simulink model "ABB_1010"  (R2024a)
settings: Solver=VariableStepAuto  StartTime=0.0  StopTime=200  RelTol=1e-3
model workspace: external: MATLAB File C:\Users\lucas\OneDrive\Documents\MATLAB\projeto final\ABB_1010_DataFile.m (data not in the file)
values from neighbouring files (symbols this model uses):
  g = 9.81    [inicializacaoAntropomorfico.m]
  I1 = [ 0.00243841  0.00000307  0.00007261    [inicializacaoAntropomorfico.m]
  I2 = [ 0.01633569  0.00000387 -0.00034405    [inicializacaoAntropomorfico.m]
  I3 = [ 0.00244760 -0.00000208  0.00000538    [inicializacaoAntropomorfico.m]
  I4 = [ 0.00245792 -0.00000008  0.00003121    [inicializacaoAntropomorfico.m]
  I5 = [ 0.00062165 -0.00000206 -0.00000303    [inicializacaoAntropomorfico.m]
  I6 = [ 0.00000357  0.00000000  0.00000000    [inicializacaoAntropomorfico.m]
  I7 = [(m7*L7^2)/12 0.00000000  0.00000000    [inicializacaoAntropomorfico.m]
  L = [L1, L2, L3, L4, L5, L6, L7]    [inicializacaoAntropomorfico.m]
  Lcm1 = [-0.00258308  0.00024508 -0.01434968]    [inicializacaoAntropomorfico.m]
  Lcm2 = [-0.02078894  0.00020016 -0.10516734]    [inicializacaoAntropomorfico.m]
  Lcm3 = [ 0.00021912  0.00015355 -0.06228290]    [inicializacaoAntropomorfico.m]
  Lcm4 = [-0.00172658 -0.00124140 -0.07369196]    [inicializacaoAntropomorfico.m]
  Lcm5 = [-0.00014110  0.00085992 -0.03825278]    [inicializacaoAntropomorfico.m]
  Lcm6 = [ 0.00002478  0.00000000 -0.00042157]    [inicializacaoAntropomorfico.m]
  Lcm7 = [ 0           0          -0.05000000]    [inicializacaoAntropomorfico.m]
  m = [m1, m2, m3, m4, m5, m6, m7]    [inicializacaoAntropomorfico.m]
  Pf = [  0.05    [inicializacaoAntropomorfico.m]
  Pi = [  0.2    [inicializacaoAntropomorfico.m]
  Raio = [0]    [inicializacaoAntropomorfico.m]
  Sentido = [0]    [inicializacaoAntropomorfico.m]
  Tipo = [1]    [inicializacaoAntropomorfico.m]
undefined symbols (not defined in the file or in its folder): smiData, X, Y, Z
libraries: sm_lib x35, nesl_utility x7
(part 3 of 16)

== matlab function ABB_1010/Dinamica1/MATLAB Function1 ==
  data: I1 parameter; L parameter; Lcm1 parameter; H output; Q input; I2 parameter; I3 parameter; I4 parameter; I5 parameter; I6 parameter; Lcm2 parameter; Lcm3 parameter; Lcm4 parameter; Lcm5 parameter; Lcm6 parameter; dQ input; m parameter; Lcm7 parameter; I7 parameter
function H = func_H(I1, L, Lcm1, Q, I2, I3, I4, I5, I6, Lcm2, Lcm3, Lcm4, Lcm5, Lcm6, dQ, m, Lcm7, I7)
%func_H
%    OUT1 = func_H(Ixx2,Ixx3,Ixx4,Ixx5,Ixx6,Ixy2,Ixy3,Ixy4,Ixy5,Ixy6,Ixz2,Ixz3,Ixz4,Ixz5,Ixz6,Iyx2,Iyx3,Iyx4,Iyx5,Iyx6,Iyy4,Iyy5,Iyy6,Iyz2,Iyz3,Iyz4,Iyz5,Iyz6,Izx2,Izx3,Izx4,Izx5,Izx6,Izy2,Izy3,Izy4,Izy5,Izy6,Izz2,Izz3,Izz4,Izz5,Izz6,Lx2,Lx3,Lxcm2,Lxcm3,Lxcm4,Lxcm5,Lxcm6,Lycm2,Lycm3,Lycm4,Lycm5,Lycm6,Lz4,Lz5,Lzcm2,Lzcm3,Lzcm4,Lzcm5,Lzcm6,Q1,Q2,Q3,Q4,Q5,Q6,dQ1,dQ2,dQ3,dQ4,dQ5,dQ6,M2,M3,M4,M5,M6)

%    This function was generated by the Symbolic Math Toolbox version 24.1.
%    30-Apr-2025 06:22:27
H   = zeros(6,1);
m1  = m(1);
m2  = m(2);
m3  = m(3);
m4  = m(4);
m5  = m(5);
m6  = m(6);
m7  = m(7);

Q1  = Q(1);
Q2  = Q(2);
Q3  = Q(3);
Q4  = Q(4);
Q5  = Q(5);
Q6  = Q(6);

dQ1  = dQ(1);
dQ2  = dQ(2);
dQ3  = dQ(3);
dQ4  = dQ(4);
dQ5  = dQ(5);
dQ6  = dQ(6);

Lz1 = L(1);
Lx2 = L(2);
Lx3 = L(3);
Lx4 = L(4);
Lz5 = L(5);
Lz6 = L(6);
Lz7 = L(7);

Lxcm1 = Lcm1(1);
Lycm1 = Lcm1(2);
Lzcm1 = Lcm1(3);

Lxcm2 = Lcm2(1);
Lycm2 = Lcm2(2);
Lzcm2 = Lcm2(3);

Lxcm3 = Lcm3(1);
Lycm3 = Lcm3(2);
Lzcm3 = Lcm3(3);

Lxcm4 = Lcm4(1);
Lycm4 = Lcm4(2);
Lzcm4 = Lcm4(3);

Lxcm5 = Lcm5(1);
Lycm5 = Lcm5(2);
Lzcm5 = Lcm5(3);

Lxcm6 = Lcm6(1);
Lycm6 = Lcm6(2);
Lzcm6 = Lcm6(3);

Lxcm7 = Lcm7(1);
Lycm7 = Lcm7(2);
Lzcm7 = Lcm7(3);

Ixx1 = I1(1,1);
Ixy1 = I1(1,2);
Ixz1 = I1(1,3);
Iyx1 = I1(2,1);
Iyy1 = I1(2,2);
Iyz1 = I1(2,3);
Izx1 = I1(3,1);
Izy1 = I1(3,2);
Izz1 = I1(3,3);

Ixx2 = I2(1,1);
Ixy2 = I2(1,2);
Ixz2 = I2(1,3);
Iyx2 = I2(2,1);
Iyy2 = I2(2,2);
Iyz2 = I2(2,3);
Izx2 = I2(3,1);
Izy2 = I2(3,2);
Izz2 = I2(3,3);

Ixx3 = I3(1,1);
Ixy3 = I3(1,2);
Ixz3 = I3(1,3);
Iyx3 = I3(2,1);
Iyy3 = I3(2,2);
Iyz3 = I3(2,3);
Izx3 = I3(3,1);
Izy3 = I3(3,2);
Izz3 = I3(3,3);

Ixx4 = I4(1,1);
Ixy4 = I4(1,2);
Ixz4 = I4(1,3);
Iyx4 = I4(2,1);
Iyy4 = I4(2,2);
Iyz4 = I4(2,3);
Izx4 = I4(3,1);
Izy4 = I4(3,2);
Izz4 = I4(3,3);

Ixx5 = I5(1,1);
Ixy5 = I5(1,2);
Ixz5 = I5(1,3);
Iyx5 = I5(2,1);
Iyy5 = I5(2,2);
Iyz5 = I5(2,3);
Izx5 = I5(3,1);
Izy5 = I5(3,2);
Izz5 = I5(3,3);

Ixx6 = I6(1,1);
Ixy6 = I6(1,2);
Ixz6 = I6(1,3);
Iyx6 = I6(2,1);
Iyy6 = I6(2,2);
Iyz6 = I6(2,3);
Izx6 = I6(3,1);
Izy6 = I6(3,2);
Izz6 = I6(3,3);

Ixx7 = I7(1,1);
Ixy7 = I7(1,2);
Ixz7 = I7(1,3);
Iyx7 = I7(2,1);
Iyy7 = I7(2,2);
Iyz7 = I7(2,3);
Izx7 = I7(3,1);
Izy7 = I7(3,2);
Izz7 = I7(3,3);


t2 = cos(Q1);
t3 = cos(Q2);
t4 = cos(Q3);
t5 = cos(Q4);
t6 = cos(Q5);
t7 = cos(Q6);
t8 = sin(Q1);
t9 = sin(Q2);
t10 = sin(Q3);
t11 = sin(Q4);
t12 = sin(Q5);
t13 = sin(Q6);
t14 = Q2+Q3;
t15 = Lx4^2;
t16 = Lxcm4^2;
t17 = Lxcm5^2;
t18 = Lxcm6^2;
t19 = Lycm4^2;
t20 = Lycm5^2;
t21 = Lycm6^2;
t22 = Lz6^2;
t23 = Lzcm5^2;
t24 = Lzcm6^2;
t25 = Q2*2.0;
t27 = Q4*2.0;
t28 = Q5*2.0;
t29 = Q6*2.0;
t30 = dQ1^2;
t31 = dQ2^2;
t32 = dQ3^2;
t33 = dQ4^2;
t34 = dQ5^2;
t35 = dQ6^2;
t36 = cos(t27);
t37 = cos(t28);
t38 = cos(t29);
t39 = t5^2;
t40 = t6^2;
t41 = t7^2;
t42 = sin(t25);
t43 = t11^2;
t44 = t12^2;
t45 = t13^2;
t46 = Lycm3*t2;
t47 = Lzcm2*t3;
t48 = cos(t14);
t49 = Lx2*t9;
t50 = Lxcm2*t9;
t51 = Lycm3*t8;
t52 = sin(t14);
t53 = t2*t5;
t54 = Lzcm3*m3*t4;
t55 = Lzcm4*m4*t4;
t56 = t2*t11;
t57 = t5*t8;
t58 = Lx3*m3*t10;
t59 = Lx3*m4*t10;
t60 = Lx3*m5*t10;
t61 = Lx3*m6*t10;
t62 = Lxcm3*m3*t10;
t63 = t8*t11;
t65 = Lx2*t2*t3;
t68 = Lzcm4*t3*t4;
t69 = Lx3*Lycm4*m4*t5;
t70 = Lx3*Lycm5*m5*t5;
t71 = Lx3*Lz6*m6*t6;
t72 = Lx4*Lzcm4*m4*t5;
t73 = Lx3*Lzcm5*m5*t6;
t74 = Lx3*Lzcm6*m6*t6;
t75 = Lxcm4*Lzcm4*m4*t5;
t76 = Lxcm5*Lzcm5*m5*t5;
t79 = Ixx4*t5*t11;
t80 = Ixx6*t5*t11;
t81 = Ixx5*t6*t12;
t82 = Ixx6*t7*t13;
t83 = Iyy4*t5*t11;
t84 = Iyy5*t5*t11;
t85 = Iyy6*t6*t12;
t86 = Iyy6*t7*t13;
t87 = Izz5*t5*t11;
t88 = Izz6*t5*t11;
t89 = Izz5*t6*t12;
t90 = Izz6*t6*t12;
t91 = Lx2*t3*t8;
t92 = Lx3*t3*t10;
t93 = Lx3*t4*t9;
t98 = Lx3*Lx4*m4*t11;
t99 = Lx3*Lx4*m5*t11;
t100 = Lx3*Lx4*m6*t11;
t101 = Lx3*Lxcm4*m4*t11;
t102 = Lx3*Lxcm5*m5*t12;
t103 = Lycm4*Lzcm4*m4*t11;
t106 = Lzcm4*t9*t10;
t110 = Lxcm6*Lz6*t5*t7;
t111 = Lxcm6*Lzcm6*t5*t7;
t112 = Lx3*Lxcm6*t7*t12;
t113 = Lycm6*Lz6*t5*t13;
t114 = Lycm6*Lzcm6*t5*t13;
t116 = t2*t3*t4;
t117 = Lx3*Lycm6*t12*t13;
t118 = Lz6*m6*t4*t6;
t119 = Lzcm5*m5*t4*t6;
t120 = Lzcm6*m6*t4*t6;
t123 = t2*t3*t10;
t124 = t2*t4*t9;
t125 = t3*t4*t8;
t127 = Lx4*m4*t5*t10;
t128 = Lx4*m5*t5*t10;
t129 = Lx4*m6*t5*t10;
t130 = Lxcm4*m4*t5*t10;
t131 = Lxcm5*m5*t4*t12;
t133 = t2*t9*t10;
t134 = t3*t8*t10;
t135 = t4*t8*t9;
t137 = Lycm4*m4*t10*t11;
t138 = Lycm5*m5*t10*t11;
t139 = t8*t9*t10;
t140 = t14*2.0;
t170 = Lx3*Lycm6*m6*t5*t7;
t172 = Lx4*Lz6*m6*t5*t6;
t174 = Lx4*Lzcm5*m5*t5*t6;
t176 = Lx4*Lzcm6*m6*t5*t6;
t187 = Lx4*t3*t5*t10;
t188 = Lx4*t4*t5*t9;
t190 = Lxcm4*t3*t5*t10;
t191 = Lxcm4*t4*t5*t9;
t199 = Lx3*Lxcm5*m5*t6*t11;
t200 = Lx4*Lxcm5*m5*t5*t12;
t201 = Lx3*Lxcm6*m6*t5*t13;
t202 = Lx3*Lxcm6*m6*t7*t11;
t205 = Lycm6*Lz6*m6*t7*t12;
t206 = Lycm5*Lzcm5*m5*t6*t11;
t208 = Lycm6*Lzcm6*m6*t7*t12;
t214 = Lycm4*t3*t10*t11;
t215 = Lycm4*t4*t9*t11;
t221 = Lx3*Lycm6*m6*t11*t13;
t223 = Lxcm5*Lycm5*m5*t11*t12;
t224 = Lxcm6*Lycm6*m6*t11*t12;
t225 = Lx3*Lz6*m6*t11*t12;
t226 = Lx3*Lzcm5*m5*t11*t12;
t227 = Lx3*Lzcm6*m6*t11*t12;
t228 = Lxcm6*Lz6*m6*t12*t13;
t229 = Lxcm6*Lzcm6*m6*t12*t13;
t235 = Lx4*Lxcm6*t5*t7*t12;
t236 = Lycm6*Lz6*t6*t7*t11;
t237 = Lycm6*Lzcm6*t6*t7*t11;
t239 = Lx4*Lycm6*t5*t12*t13;
t240 = Lxcm6*Lz6*t6*t11*t13;
t241 = Lxcm6*Lzcm6*t6*t11*t13;
t247 = Lxcm5*m5*t5*t6*t10;
t248 = Lxcm6*m6*t4*t7*t12;
t256 = Lycm6*m6*t7*t10*t11;
t257 = Lycm6*m6*t4*t12*t13;
t258 = Lz6*m6*t5*t10*t12;
t259 = Lzcm5*m5*t5*t10*t12;
t260 = Lzcm6*m6*t5*t10*t12;
t267 = Lxcm6*m6*t10*t11*t13;
t278 = Lx4*Lxcm4*m4*t5*t11*2.0;
t279 = Lz6*Lzcm6*m6*t5*t11*2.0;
t280 = Lz6*Lzcm6*m6*t6*t12*2.0;
t281 = m4*t5*t11*t15;
t282 = m5*t5*t11*t15;
t283 = m6*t5*t11*t15;
t284 = m4*t5*t11*t16;
t285 = m5*t6*t12*t17;
t286 = m6*t5*t11*t18;
t287 = m6*t7*t13*t18;
t288 = m4*t5*t11*t19;
t289 = m5*t5*t11*t20;
t290 = m6*t6*t12*t21;
t291 = m6*t7*t13*t21;
t292 = m6*t5*t11*t22;
t293 = m6*t6*t12*t22;
t294 = m5*t5*t11*t23;
t295 = m5*t6*t12*t23;
t296 = m6*t5*t11*t24;
t297 = m6*t6*t12*t24;
t352 = Lx4*Lxcm6*m6*t5*t7*t11;
t374 = Lx4*Lycm6*m6*t5*t11*t13;
t420 = Lycm6*m6*t5*t6*t10*t13;
t434 = Lx4*Lxcm5*m5*t5*t6*t11*2.0;
t436 = Lx4*Lz6*m6*t5*t11*t12*2.0;
t437 = Lx4*Lzcm5*m5*t5*t11*t12*2.0;
t438 = Lx4*Lzcm6*m6*t5*t11*t12*2.0;
t453 = Lxcm6*m6*t5*t6*t7*t10;
t590 = Lxcm6*Lycm6*m6*t5*t7*t11*t13*2.0;
t591 = Lxcm6*Lycm6*m6*t6*t7*t12*t13*2.0;
t679 = Lxcm6*Lycm6*m6*t5*t6*t7*t11*t13*4.0;
t64 = Lzcm3*t48;
t66 = Lycm4*t53;
t67 = Lycm5*t53;
t77 = Lx3*t52;
t78 = Lxcm3*t52;
t94 = Lx4*t56;
t95 = Lxcm4*t56;
t96 = Lycm4*t57;
t97 = Lycm5*t57;
t104 = Lx4*t63;
t105 = Lxcm4*t63;
t107 = -t47;
t108 = -t51;
t109 = t52^2;
t115 = t6*t48;
t121 = t12*t48;
t122 = t6*t52;
t126 = t6*t56;
t132 = t12*t52;
t136 = t12*t56;
t141 = -t53;
t142 = -t54;
t143 = -t55;
t144 = -t63;
t146 = -t65;
t147 = -t68;
t148 = -t76;
t149 = -t79;
t150 = -t87;
t151 = -t88;
t152 = -t89;
t153 = -t90;
t155 = -t103;
t156 = sin(t140);
t159 = Lx4*Lycm4*m4*t36;
t160 = Lx4*Lycm5*m5*t36;
t161 = Lxcm4*Lycm4*m4*t36;
t162 = Lxcm6*Lycm6*m6*t38;
t163 = Lxcm5*Lzcm5*m5*t37;
t164 = Lx3*t2*t48;
t168 = Lx3*t116;
t169 = Lxcm3*t116;
t171 = t5*t71;
t173 = t5*t73;
t175 = t5*t74;
t177 = m6*t110;
t178 = m6*t111;
t179 = Lx3*t8*t48;
t180 = Lx4*t5*t52;
t182 = t5*t81;
t183 = t5*t85;
t186 = Lx3*t125;
t189 = Lxcm3*t125;
t193 = Lycm6*t7*t57;
t194 = Lzcm3*t123;
t195 = Lzcm3*t124;
t196 = Lzcm4*t123;
t197 = Lzcm4*t124;
t198 = t5*t102;
t203 = m6*t112;
t204 = m6*t113;
t207 = m6*t114;
t209 = Lycm5*t11*t52;
t210 = Lx3*t133;
t211 = Lxcm3*t133;
t212 = Lxcm5*t6*t63;
t213 = Lxcm6*t13*t57;
t216 = Lzcm3*t134;
t217 = Lzcm3*t135;
t218 = Lzcm4*t134;
t219 = Lzcm4*t135;
t222 = m6*t117;
t230 = Lx3*t139;
t231 = Lxcm3*t139;
t232 = Lz6*t12*t63;
t233 = Lzcm5*t12*t63;
t234 = Lzcm6*t12*t63;
t244 = t7*t11*t48;
t246 = t3*t4*t57;
t251 = t11*t13*t48;
t252 = t7*t11*t52;
t262 = t11*t13*t52;
t264 = t9*t10*t57;
t265 = -t110;
t266 = -t111;
t268 = t9*t10*t63;
t269 = -t112;
t270 = -t118;
t271 = -t119;
t272 = -t120;
t274 = -t133;
t275 = -t137;
t276 = -t138;
t277 = -t139;
t298 = Lx4*Lycm6*m6*t7*t39;
t299 = Lxcm5*Lycm5*m5*t6*t39;
t300 = Lxcm6*Lycm6*m6*t6*t39;
t301 = Lx4*Lz6*m6*t6*t39;
t302 = Lx4*Lzcm5*m5*t6*t39;
t303 = Lx4*Lzcm6*m6*t6*t39;
t304 = Lxcm6*Lz6*m6*t7*t40;
t305 = Lxcm6*Lzcm6*m6*t7*t40;
t306 = Ixx5*t5*t11*t40;
t307 = t39*t81;
t308 = t41*t80;
t309 = Ixx6*t6*t12*t41;
t310 = t39*t82;
t311 = t40*t82;
t312 = Iyy6*t5*t11*t40;
t313 = Iyy6*t5*t11*t41;
t314 = t39*t85;
t315 = t41*t85;
t316 = t39*t86;
t317 = t40*t86;
t318 = t40*t87;
t319 = t39*t89;
t320 = t40*t88;
t321 = t39*t90;
t322 = Lx4*Lxcm5*m5*t12*t39;
t323 = Lx4*Lxcm6*m6*t13*t39;
t324 = Lx4*Lycm6*m6*t7*t43;
t325 = Lxcm5*Lycm5*m5*t6*t43;
t326 = Lxcm6*Lycm6*m6*t6*t43;
t327 = Lxcm6*Lz6*m6*t7*t44;
t328 = Lxcm6*Lzcm6*m6*t7*t44;
t329 = Lycm6*Lz6*m6*t13*t40;
t330 = Lycm5*Lzcm5*m5*t12*t39;
t331 = Lycm6*Lzcm6*m6*t13*t40;
t332 = Lx4*Lxcm6*m6*t13*t43;
t333 = Lycm6*Lz6*m6*t13*t44;
t334 = Lycm5*Lzcm5*m5*t12*t43;
t335 = Lycm6*Lzcm6*m6*t13*t44;
t336 = Lx4*t3*t4*t53;
t337 = Lxcm4*t3*t4*t53;
t338 = t6*t170;
t346 = Lycm4*t3*t4*t56;
t347 = Lycm5*t3*t4*t56;
t348 = Lx2*t247;
t349 = t6*t201;
t351 = t6*t202;
t353 = m6*t235;
t354 = m6*t236;
t355 = t6*t205;
t356 = t5*t206;
t357 = m6*t237;
t358 = t6*t208;
t365 = Lx4*t9*t10*t53;
t367 = Lxcm5*t12*t123;
t368 = Lxcm5*t12*t124;
t369 = Lxcm6*t6*t7*t63;
t373 = t6*t221;
t375 = m6*t239;
t376 = t5*t223;
t377 = t5*t224;
t378 = Lx2*t258;
t379 = Lx2*t259;
t380 = Lx2*t260;
t381 = m6*t240;
t382 = t6*t228;
t383 = m6*t241;
t384 = t6*t229;
t387 = t11*t12*t82;
t388 = t11*t12*t86;
t391 = Lycm4*t9*t10*t56;
t392 = Lycm5*t9*t10*t56;
t407 = -t200;
t408 = -t206;
t412 = -t214;
t413 = -t215;
t414 = -t221;
t415 = -t224;
t423 = -t235;
t425 = t40*t76*2.0;
t428 = -t256;
t429 = -t257;
t433 = -t267;
t435 = t5*t280;
t439 = t5*t285;
t440 = t5*t290;
t441 = t5*t293;
t442 = t5*t295;
t443 = t5*t297;
t445 = -t285;
t446 = -t286;
t447 = -t288;
t448 = -t289;
t449 = -t290;
t454 = Lx4*Lycm6*m6*t12*t13*t39;
t455 = t39*t228;
t456 = t39*t229;
t457 = t43*t205;
t458 = t43*t208;
t459 = t43*t228;
t460 = t43*t229;
t482 = Lycm6*t3*t4*t7*t56;
t486 = Lx2*t453;
t492 = Lxcm5*t6*t9*t10*t53;
t493 = Lxcm6*t3*t4*t13*t56;
t494 = Lxcm6*t7*t12*t123;
t495 = Lxcm6*t7*t12*t124;
t497 = Lx2*t420;
t502 = t7*t12*t13*t80;
t505 = Lycm6*t7*t9*t10*t56;
t506 = Lycm6*t12*t13*t123;
t507 = Lycm6*t12*t13*t124;
t508 = Lz6*t9*t10*t12*t53;
t509 = Lzcm5*t9*t10*t12*t53;
t510 = Lzcm6*t9*t10*t12*t53;
t513 = Lxcm6*t9*t10*t13*t56;
t519 = Lxcm6*Lycm6*m6*t39*t41;
t520 = Lxcm6*Lycm6*m6*t40*t41;
t521 = Lxcm5*Lzcm5*m5*t39*t40;
t530 = Lxcm6*Lycm6*m6*t39*t45;
t531 = Lxcm6*Lycm6*m6*t40*t45;
t532 = Lxcm5*Lzcm5*m5*t39*t44;
t539 = -t374;
t560 = Lx4*Lxcm6*m6*t7*t12*t39;
t561 = t39*t205;
t562 = t39*t208;
t563 = t6*t45*t80;
t564 = t6*t43*t82;
t565 = Iyy6*t5*t6*t11*t45;
t566 = t6*t43*t86;
t567 = t41*t224*2.0;
t568 = m5*t5*t11*t17*t40;
t569 = t39*t285;
t570 = t41*t286;
t571 = m6*t6*t12*t18*t41;
t572 = t39*t287;
t573 = t40*t287;
t574 = m6*t5*t11*t21*t40;
t575 = m6*t5*t11*t21*t41;
t576 = t39*t290;
t577 = t41*t290;
t578 = t39*t291;
t579 = t40*t291;
t580 = t40*t292;
t581 = t39*t293;
t582 = t40*t294;
t583 = t39*t295;
t584 = t40*t296;
t585 = t39*t297;
t586 = -t420;
t588 = t6*t352*2.0;
t589 = t6*t374*2.0;
t592 = t6*t11*t12*t76*2.0;
t593 = t11*t12*t287;
t594 = t11*t12*t291;
t605 = t40*t279;
t611 = Lxcm6*t6*t7*t9*t10*t53;
t634 = -t590;
t648 = Ixx4*t39*t48*t52;
t650 = Iyy4*t43*t48*t52;
t651 = Iyy5*t43*t48*t52;
t663 = Lz6*Lzcm6*m6*t5*t11*t40*-2.0;
t664 = Lz6*Lzcm6*m6*t6*t12*t39*-2.0;
t665 = Lycm6*t3*t4*t6*t13*t53;
t678 = t5*t591;
t688 = t123+t124;
t690 = t134+t135;
t700 = t6*t43*t287;
t701 = m6*t5*t6*t11*t21*t45;
t702 = t6*t43*t291;
t703 = -t679;
t740 = Lxcm6*Lycm6*m6*t5*t7*t11*t13*t40*-2.0;
t145 = -t64;
t154 = -t96;
t157 = -t104;
t158 = -t105;
t165 = Lz6*t115;
t166 = Lzcm5*t115;
t167 = Lzcm6*t115;
t181 = Lxcm5*t121;
t192 = Lxcm5*t126;
t220 = Lzcm5*t136;
t238 = t5*t115;
t242 = t5*t121;
t243 = t5*t122;
t245 = t7*t121;
t249 = t8*t122;
t250 = t5*t132;
t253 = t13*t121;
t254 = t7*t132;
t261 = t8*t132;
t263 = t13*t132;
t341 = Lz6*t2*t122;
t342 = Lzcm5*t2*t122;
t343 = Lzcm6*t2*t122;
t344 = Lx4*t246;
t345 = Lxcm4*t246;
t350 = t5*t203;
t359 = Lycm6*t252;
t372 = t5*t222;
t386 = Lxcm6*t262;
t389 = Lx4*t264;
t390 = Lxcm4*t264;
t394 = Lycm4*t268;
t395 = Lycm5*t268;
t396 = -t164;
t400 = -t171;
t401 = -t173;
t402 = -t175;
t403 = -t177;
t404 = -t178;
t405 = t5*t152;
t406 = t5*t153;
t409 = -t209;
t410 = -t210;
t411 = -t211;
t416 = -t230;
t417 = -t231;
t419 = t12*t246;
out1 = ft_1({Ixx2,Ixx3,Ixx5,Ixx6,Iyy6,Izz2,Izz3,Izz4,Izz5,Izz6,Lx2,Lx3,Lx4,Lxcm2,Lxcm3,Lxcm4,Lxcm5,Lxcm6,Lycm2,Lycm3,Lycm4,Lycm5,Lycm6,Lz6,Lzcm2,Lzcm3,Lzcm4,Lzcm5,Lzcm6,m2,m3,m4,m5,m6,t10,t100,t101,t102,t104,t106,t107,t108,t109,t11,t113,t114,t115,t116,t117,t118,t119,t12,t120,t121,t122,t125,t126,t127,t128,t129,t13,t130,t131,t132,t136,t141,t142,t143,t144,t145,t146,t147,t148,t149,t150,t151,t152,t153,t154,t155,t156,t157,t158,t159,t160,t161,t162,t163,t165,t166,t167,t168,t169,t170,t172,t174,t176,t177,t178,t179,t180,t181,t182,t183,t186,t187,t188,t189,t190,t191,t192,t193,t194,t195,t196,t197,t198,t199,t2,t200,t201,t202,t203,t204,t205,t206,t207,t208,t212,t213,t216,t217,t218,t219,t220,t222,t223,t224,t225,t226,t227,t228,t229,t232,t233,t234,t236,t237,t238,t239,t240,t241,t242,t243,t244,t245,t246,t247,t248,t249,t250,t251,t252,t253,t254,t256,t257,t258,t259,t260,t261,t262,t263,t264,t265,t266,t268,t269,t270,t271,t272,t274,t275,t276,t277,t278,t279,t280,t281,t282,t283,t284,t285,t286,t287,t288,t289,t290,t291,t292,t293,t294,t295,t296,t297,t298,t299,t3,t30,t300,t301,t302,t303,t304,t305,t306,t307,t308,t309,t31,t310,t311,t312,t313,t314,t315,t316,t317,t318,t319,t32,t320,t321,t322,t323,t324,t325,t326,t327,t328,t329,t33,t330,t331,t332,t333,t334,t335,t336,t337,t338,t34,t341,t342,t343,t344,t345,t346,t347,t348,t349,t35,t350,t351,t352,t353,t354,t355,t356,t357,t358,t359,t365,t367,t368,t369,t372,t373,t374,t375,t376,t377,t378,t379,t380,t381,t382,t383,t384,t386,t387,t388,t389,t39,t390,t391,t392,t394,t395,t396,t4,t40,t400,t401,t402,t403,t404,t405,t406,t407,t408,t409,t41,t410,t411,t412,t413,t414,t415,t416,t417,t419,t42,t423,t425,t428,t429,t43,t433,t434,t435,t436,t437,t438,t439,t44,t440,t441,t442,t443,t445,t446,t447,t448,t449,t45,t453,t454,t455,t456,t457,t458,t459,t46,t460,t482,t486,t49,t492,t493,t494,t495,t497,t5,t50,t502,t505,t506,t507,t508,t509,t510,t513,t519,t52,t520,t521,t53,t530,t531,t532,t539,t54,t55,t56,t560,t561,t562,t563,t564,t565,t566,t567,t568,t569,t57,t570,t571,t572,t573,t574,t575,t576,t577,t578,t579,t58,t580,t581,t582,t583,t584,t585,t586,t588,t589,t59,t591,t592,t593,t594,t6,t60,t605,t61,t611,t62,t63,t634,t648,t65,t650,t651,t66,t663,t664,t665,t67,t678,t688,t69,t690,t7,t70,t700,t701,t702,t703,t71,t72,t73,t74,t740,t75,t76,t77,t78,t79,t8,t80,t81,t82,t83,t84,t85,t86,t87,t88,t89,t9,t90,t91,t92,t93,t94,t95,t97,t98,t99});
end
function out1 = ft_1(ct)
[Ixx2,Ixx3,Ixx5,Ixx6,Iyy6,Izz2,Izz3,Izz4,Izz5,Izz6,Lx2,Lx3,Lx4,Lxcm2,Lxcm3,Lxcm4,Lxcm5,Lxcm6,Lycm2,Lycm3,Lycm4,Lycm5,Lycm6,Lz6,Lzcm2,Lzcm3,Lzcm4,Lzcm5,Lzcm6,m2,m3,m4,m5,m6,t10,t100,t101,t102,t104,t106,t107,t108,t109,t11,t113,t114,t115,t116,t117,t118,t119,t12,t120,t121,t122,t125,t126,t127,t128,t129,t13,t130,t131,t132,t136,t141,t142,t143,t144,t145,t146,t147,t148,t149,t150,t151,t152,t153,t154,t155,t156,t157,t158,t159,t160,t161,t162,t163,t165,t166,t167,t168,t169,t170,t172,t174,t176,t177,t178,t179,t180,t181,t182,t183,t186,t187,t188,t189,t190,t191,t192,t193,t194,t195,t196,t197,t198,t199,t2,t200,t201,t202,t203,t204,t205,t206,t207,t208,t212,t213,t216,t217,t218,t219,t220,t222,t223,t224,t225,t226,t227,t228,t229,t232,t233,t234,t236,t237,t238,t239,t240,t241,t242,t243,t244,t245,t246,t247,t248,t249,t250,t251,t252,t253,t254,t256,t257,t258,t259,t260,t261,t262,t263,t264,t265,t266,t268,t269,t270,t271,t272,t274,t275,t276,t277,t278,t279,t280,t281,t282,t283,t284,t285,t286,t287,t288,t289,t290,t291,t292,t293,t294,t295,t296,t297,t298,t299,t3,t30,t300,t301,t302,t303,t304,t305,t306,t307,t308,t309,t31,t310,t311,t312,t313,t314,t315,t316,t317,t318,t319,t32,t320,t321,t322,t323,t324,t325,t326,t327,t328,t329,t33,t330,t331,t332,t333,t334,t335,t336,t337,t338,t34,t341,t342,t343,t344,t345,t346,t347,t348,t349,t35,t350,t351,t352,t353,t354,t355,t356,t357,t358,t359,t365,t367,t368,t369,t372,t373,t374,t375,t376,t377,t378,t379,t380,t381,t382,t383,t384,t386,t387,t388,t389,t39,t390,t391,t392,t394,t395,t396,t4,t40,t400,t401,t402,t403,t404,t405,t406,t407,t408,t409,t41,t410,t411,t412,t413,t414,t415,t416,t417,t419,t42,t423,t425,t428,t429,t43,t433,t434,t435,t436,t437,t438,t439,t44,t440,t441,t442,t443,t445,t446,t447,t448,t449,t45,t453,t454,t455,t456,t457,t458,t459,t46,t460,t482,t486,t49,t492,t493,t494,t495,t497,t5,t50,t502,t505,t506,t507,t508,t509,t510,t513,t519,t52,t520,t521,t53,t530,t531,t532,t539,t54,t55,t56,t560,t561,t562,t563,t564,t565,t566,t567,t568,t569,t57,t570,t571,t572,t573,t574,t575,t576,t577,t578,t579,t58,t580,t581,t582,t583,t584,t585,t586,t588,t589,t59,t591,t592,t593,t594,t6,t60,t605,t61,t611,t62,t63,t634,t648,t65,t650,t651,t66,t663,t664,t665,t67,t678,t688,t69,t690,t7,t70,t700,t701,t702,t703,t71,t72,t73,t74,t740,t75,t76,t77,t78,t79,t8,t80,t81,t82,t83,t84,t85,t86,t87,t88,t89,t9,t90,t91,t92,t93,t94,t95,t97,t98,t99] = ct{:};
t421 = t6*t264;
t422 = t12*t264;
t427 = t3*t4*t144;
t430 = -t262;
t432 = -t264;
t452 = t6*t246;
t461 = -t300;
t462 = -t301;
t463 = -t302;
t464 = -t303;
t466 = -t306;
t467 = -t307;
t468 = -t308;
t469 = -t310;
t470 = -t312;
t471 = -t314;
t472 = -t315;
t473 = -t317;
t474 = -t324;
t475 = -t325;
t476 = -t327;
t477 = -t328;
t478 = -t329;
t479 = -t331;
t487 = t5*t354;
t488 = t5*t357;
t489 = -t332;
t490 = -t334;
t498 = t5*t381;
t499 = t11*t12*t177;
t500 = t5*t383;
t501 = t11*t12*t178;
t503 = t5*t388;
t511 = t11*t12*t204;
t512 = t11*t12*t207;
t515 = Lx4*t3*t4*t141;
t522 = -t346;
t523 = -t353;
t524 = -t354;
t525 = -t355;
t526 = -t357;
t527 = -t358;
t533 = Lx4*t9*t10*t141;
t534 = Lxcm4*t9*t10*t141;
t538 = -t373;
t540 = -t376;
t541 = -t381;
t542 = -t382;
t543 = -t383;
t544 = -t384;
t547 = -t387;
t550 = -t392;
t551 = Lycm6*t6*t13*t144;
t552 = t6*t298;
t554 = t5*t309;
t555 = t6*t310;
t556 = t6*t313;
t557 = t41*t183;
t558 = t6*t316;
t559 = t6*t323;
t595 = -t439;
t596 = -t440;
t597 = (Ixx3*t156)./2.0;
t598 = (Izz3*t156)./2.0;
t599 = (Izz4*t156)./2.0;
t601 = t40*t177*2.0;
t602 = t40*t178*2.0;
t603 = t40*t204*2.0;
t604 = t40*t207*2.0;
t608 = -t454;
t609 = -t457;
t610 = -t458;
t612 = -t459;
t613 = -t460;
t615 = Lxcm5*t3*t4*t6*t141;
t616 = t39*t304;
t617 = t39*t305;
t618 = Lz6*t3*t4*t12*t141;
t619 = Lzcm5*t3*t4*t12*t141;
t620 = Lzcm6*t3*t4*t12*t141;
t621 = t40*t308;
t622 = t39*t309;
t624 = t41*t312;
t625 = t41*t314;
t626 = t40*t316;
t628 = t39*t327;
t629 = t39*t328;
t630 = t39*t329;
t631 = t39*t331;
t632 = -t497;
t633 = -t589;
t636 = t39*t333;
t637 = t39*t335;
t639 = -t505;
t640 = -t506;
t641 = -t507;
t644 = -t513;
t646 = -t520;
t647 = -t521;
t649 = -t530;
t652 = t39*t355;
t653 = t39*t358;
t654 = t39*t382;
t655 = t39*t384;
t666 = -t565;
t667 = -t566;
t668 = -t571;
t669 = -t573;
t670 = -t575;
t671 = -t578;
t672 = -t580;
t673 = -t581;
t674 = -t582;
t675 = -t583;
t676 = -t584;
t677 = -t585;
t685 = t5*t594;
t686 = t41*t300*2.0;
t687 = t41*t326*2.0;
t689 = -t594;
t691 = t49+t50+t107;
t692 = t41*t377*2.0;
t693 = t6*t570;
t695 = t6*t572;
t697 = t41*t440;
t698 = t6*t578;
t704 = Lycm6*t6*t9*t10*t13*t141;
t715 = -t648;
t716 = t40*t519;
t717 = -t650;
t718 = -t651;
t721 = Lxcm6*t3*t4*t6*t7*t141;
t722 = t40*t570;
t723 = t39*t571;
t724 = t40*t572;
t725 = t41*t574;
t730 = t7*t12*t13*t446;
t732 = t7*t12*t13*t300*2.0;
t733 = t116+t274;
t734 = t125+t277;
t738 = t6*t45*t446;
t739 = -t700;
t742 = t6*t688;
t743 = t12*t688;
t744 = t6*t690;
t746 = t12*t690;
t748 = t39*t41*t449;
t835 = t92+t93+t106+t147+t187+t188+t190+t191+t412+t413;
t856 = t58+t59+t60+t61+t62+t127+t128+t129+t130+t131+t142+t143+t247+t248+t258+t259+t260+t270+t271+t272+t275+t276+t428+t429+t433+t453+t586;
t339 = Lxcm5*t243;
t340 = Lxcm6*t245;
t360 = Lycm6*t253;
t361 = Lz6*t250;
t362 = Lzcm5*t249;
t363 = Lzcm5*t250;
t364 = Lzcm6*t250;
t385 = Lxcm5*t261;
t397 = -t165;
t398 = -t166;
t399 = -t167;
t418 = t13*t243;
t424 = -t238;
t426 = -t250;
t431 = -t263;
t450 = t13*t238;
t451 = t7*t243;
t481 = Lxcm5*t452;
t496 = Lzcm5*t419;
t504 = Lxcm5*t421;
t514 = Lzcm5*t422;
t516 = -t341;
t517 = -t342;
t518 = -t343;
t528 = -t359;
t535 = Lycm4*t427;
t536 = Lycm5*t427;
t537 = -t372;
t546 = -t386;
t548 = -t389;
t549 = -t390;
t587 = -t422;
t635 = -t503;
t642 = -t511;
t643 = -t512;
t656 = -t597;
t658 = t6*t468;
t659 = t6*t469;
t660 = -t557;
t661 = -t603;
t662 = -t604;
t680 = t6*t499*2.0;
t681 = t6*t501*2.0;
t682 = t6*t511*2.0;
t683 = t6*t512*2.0;
t707 = -t616;
t708 = -t617;
t709 = t40*t468;
t710 = -t622;
t711 = t40*t469;
t712 = -t687;
t713 = -t636;
t714 = -t637;
t720 = -t692;
t728 = t121+t243;
t729 = t122+t242;
t735 = t5*t668;
t736 = t6*t670;
t737 = t6*t671;
t741 = -t732;
t745 = t40*t649;
t747 = -t725;
t749 = t40*t671;
t750 = Lx3*t733;
t753 = Lx3*t734;
t756 = t5*t733;
t757 = t11*t733;
t758 = t5*t734;
t759 = t11*t734;
t760 = t77+t78+t145;
t763 = t56+t246+t432;
t765 = t53+t268+t427;
t805 = -t13*(t126-t261-t421+t452);
t807 = t7*(t126-t261-t421+t452);
t825 = t46+t91+t186+t189+t216+t217+t416+t417;
t828 = t65+t108+t168+t169+t194+t195+t410+t411;
t837 = t49+t835;
t851 = t65+t154+t157+t158+t168+t196+t197+t336+t337+t391+t410+t522+t533+t534;
t480 = Lxcm6*t451;
t491 = Lycm6*t418;
t529 = -t360;
t545 = -t385;
t600 = t7*t424;
t638 = -t504;
t645 = -t514;
t705 = -t682;
t706 = -t683;
t751 = t115+t426;
t752 = t132+t424;
t754 = t7*t728;
t755 = t13*t728;
t761 = t49+t760;
t762 = t57+t757;
t764 = t56+t758;
t768 = Lx4*t763;
t773 = t13*t765;
t777 = t7*t765;
t778 = -Lx4*(t63-t756);
t783 = t252+t253+t418;
t787 = -t12*(t63-t756);
t789 = -t7*(t53-t759);
t790 = Lycm5*(t53-t759);
t792 = t244+t431+t450;
t793 = t245+t430+t451;
t795 = t6*(t63-t756);
t796 = t7*(t53-t759);
t800 = t136+t249+t419+t587;
t826 = t77+t180+t181+t339+t363+t398+t409;
t848 = t66+t91+t94+t95+t186+t218+t219+t344+t345+t394+t416+t535+t548+t549;
t853 = t97+t104+t146+t212+t233+t347+t365+t367+t368+t396+t492+t509+t515+t517+t550+t615+t619;
t860 = t104+t146+t193+t213+t232+t234+t365+t369+t396+t482+t493+t494+t495+t508+t510+t515+t516+t518+t551+t611+t618+t620+t639+t640+t641+t644+t665+t704+t721;
t627 = -t491;
t766 = Lx4*t762;
t767 = Lycm5*t762;
t769 = Lx4*t764;
t772 = t12*t764;
t774 = t7*t762;
t775 = t6*t764;
t776 = t13*t762;
t782 = t252+t755;
t791 = t251+t254+t600;
t797 = Ixx5*t728*t752;
t798 = Izz5*t729*t751;
t799 = Izz6*t729*t751;
t801 = Lz6*t800;
t802 = Lzcm6*t800;
t812 = t742+t787;
t817 = t743+t795;
t827 = Iyy6*t783*t792;
t831 = t49+t826;
t832 = t777+t805;
t834 = t773+t807;
t852 = t67+t91+t94+t179+t192+t220+t344+t362+t395+t481+t496+t536+t545+t548+t638+t645;
t779 = -t767;
t788 = -t775;
t806 = t744+t772;
t813 = Lz6*t812;
t814 = Lzcm5*t812;
t815 = Lzcm6*t812;
t820 = Lxcm5*t817;
t822 = t13*t817;
t823 = t7*t817;
t829 = Ixx6*t791*t793;
t830 = -t827;
t833 = Lycm6*t832;
t836 = Lxcm6*t834;
t849 = t77+t180+t340+t361+t364+t397+t399+t480+t528+t529+t546+t627;
t808 = t746+t788;
t809 = Lz6*t806;
t810 = Lzcm5*t806;
t811 = Lzcm6*t806;
t824 = -t820;
t838 = t776+t823;
t847 = -Lycm6*(t774-t822);
t850 = t49+t849;
t857 = t91+t179+t768+t801+t802+t833+t836;
t816 = Lxcm5*t808;
t818 = t7*t808;
t819 = t13*t808;
t843 = Lxcm6*t838;
t855 = t65+t750+t778+t779+t814+t824;
t821 = -t816;
t840 = Lxcm6*(t818-t13*(t53-t759));
t842 = t796+t819;
t846 = -t843;
t844 = -t840;
t845 = Lycm6*t842;
t854 = t91+t753+t769+t790+t810+t821;
t859 = t65+t750+t778+t813+t815+t846+t847;
t858 = t91+t753+t769+t809+t811+t844+t845;
et1 = Lycm3*t9*t31*t54+Lycm3*t9*t32*t54-Lycm3*t9*t31*t58-Lycm3*t9*t32*t58-Lycm3*t9*t31*t62-Lycm3*t9*t32*t62+t3*t4*t31*t69+t3*t4*t31*t70+t3*t4*t32*t69+t3*t4*t32*t70-t3*t4*t33*t69-t3*t4*t33*t70+t3*t4*t31*t80+t3*t4*t31*t83+t3*t4*t31*t84+t3*t4*t32*t83+t3*t4*t32*t84+t9*t10*t31*t79-t9*t10*t31*t80+t9*t10*t32*t79-t9*t10*t31*t83-t9*t10*t31*t84-t9*t10*t32*t83-t9*t10*t32*t84+t3*t4*t31*t98+t3*t4*t31*t99+t3*t4*t32*t98+t9*t10*t31*t87+t3*t4*t31*t100+t3*t4*t32*t99-t3*t4*t33*t98+t9*t10*t31*t88+t3*t4*t31*t101+t3*t4*t32*t100;
et2 = -t3*t4*t33*t99+t3*t4*t32*t101-t3*t4*t33*t100-t3*t4*t33*t101+t3*t4*t31*t149+t3*t4*t31*t150+t3*t4*t32*t149+t3*t4*t31*t151+t3*t4*t31*t170+t3*t4*t32*t170-t3*t4*t33*t170-t3*t4*t35*t170+t3*t4*t31*t199+t3*t4*t32*t199+t3*t4*t31*t201-t3*t4*t33*t199+t3*t4*t32*t201-t3*t4*t34*t199-t3*t4*t33*t201-t3*t4*t31*t205-t3*t4*t35*t201-t3*t4*t31*t208+t3*t4*t34*t205-t3*t4*t35*t205+t3*t4*t34*t208-t3*t4*t35*t208+t9*t10*t31*t205+t9*t10*t31*t208-t9*t10*t34*t205+t9*t10*t35*t205-t9*t10*t34*t208+t9*t10*t35*t208+t3*t4*t31*t225+t3*t4*t31*t226;
et3 = t3*t4*t32*t225+t3*t4*t31*t227+t3*t4*t32*t226-t3*t4*t33*t225-t3*t4*t31*t228+t3*t4*t32*t227-t3*t4*t33*t226-t3*t4*t34*t225-t3*t4*t31*t229-t3*t4*t33*t227-t3*t4*t34*t226-t3*t4*t34*t227+t3*t4*t34*t228+t3*t4*t34*t229-t3*t4*t35*t228-t3*t4*t35*t229+t9*t10*t31*t228+t9*t10*t31*t229-t9*t10*t34*t228-t9*t10*t34*t229+t9*t10*t35*t228+t9*t10*t35*t229+t3*t4*t31*t278+t3*t4*t31*t279+t3*t4*t32*t278+t3*t4*t31*t281+t3*t4*t31*t282+t3*t4*t32*t281+t3*t4*t31*t283+t3*t4*t32*t282+t3*t4*t31*t284+t3*t4*t32*t283+t3*t4*t32*t284+t3*t4*t31*t292;
et4 = -t9*t10*t31*t281+t3*t4*t31*t294-t9*t10*t31*t282-t9*t10*t32*t281-t9*t10*t31*t283-t9*t10*t32*t282+t3*t4*t31*t296-t9*t10*t31*t284-t9*t10*t32*t283-t9*t10*t32*t284+t3*t4*t31*t298*2.0+t9*t10*t31*t286+t3*t4*t31*t299*2.0+t3*t4*t32*t298-t3*t4*t31*t300*2.0+t3*t4*t32*t299+t9*t10*t31*t288+t9*t10*t31*t289+t9*t10*t32*t288+t9*t10*t32*t289-t9*t10*t31*t292-t9*t10*t31*t294-t9*t10*t31*t296-t9*t10*t31*t298*2.0-t9*t10*t31*t299*2.0-t9*t10*t32*t298+t9*t10*t31*t300*2.0-t9*t10*t32*t299+t3*t4*t31*t313+t3*t4*t32*t313+t3*t4*t31*t318+t9*t10*t31*t306+t9*t10*t32*t306;
et5 = t3*t4*t31*t320+t9*t10*t31*t308+t3*t4*t31*t323*2.0+t3*t4*t32*t323+t9*t10*t31*t312-t9*t10*t31*t313-t9*t10*t32*t313+t3*t4*t31*t330*2.0+t3*t4*t32*t330-t9*t10*t31*t323*2.0-t9*t10*t32*t323+t9*t10*t32*t324+t9*t10*t32*t325-t9*t10*t31*t330*2.0-t9*t10*t32*t330+t9*t10*t32*t332+t9*t10*t32*t334+t3*t4*t31*t351+t3*t4*t32*t351-t3*t4*t33*t351-t3*t4*t34*t351-t3*t4*t35*t351+t3*t4*t33*t373+t3*t4*t34*t373+t3*t4*t35*t373+t3*t4*t31*t434+t3*t4*t32*t434+t3*t4*t31*t436+t3*t4*t31*t437+t3*t4*t32*t436+t3*t4*t31*t438+t3*t4*t32*t437+t3*t4*t32*t438+t3*t4*t31*t446+t3*t4*t31*t447+t3*t4*t31*t448;
et6 = t3*t4*t32*t447+t3*t4*t32*t448+t3*t4*t31*t455*2.0+t3*t4*t31*t456*2.0+t3*t4*t32*t455+t3*t4*t32*t456+t3*t4*t31*t466+t3*t4*t32*t466-t9*t10*t31*t455*2.0+t3*t4*t31*t468-t9*t10*t31*t456*2.0-t9*t10*t32*t455-t9*t10*t32*t456+t3*t4*t31*t470+t9*t10*t32*t457+t9*t10*t32*t458+t9*t10*t32*t459+t9*t10*t32*t460+t3*t4*t32*t474+t3*t4*t32*t475+t3*t4*t32*t489+t3*t4*t32*t490+t3*t4*t31*t538+t3*t4*t32*t538-t3*t4*t31*t555*2.0+t3*t4*t31*t558*2.0+t3*t4*t32*t558+t3*t4*t31*t561*2.0+t3*t4*t31*t562*2.0+t3*t4*t32*t561+t3*t4*t32*t562+t3*t4*t32*t564+t9*t10*t31*t555*2.0+t3*t4*t31*t568+t9*t10*t32*t555+t3*t4*t32*t568;
et7 = t3*t4*t31*t570-t9*t10*t31*t558*2.0-t9*t10*t32*t558-t9*t10*t31*t561*2.0+t3*t4*t31*t574-t9*t10*t31*t562*2.0-t9*t10*t32*t561-t9*t10*t32*t562-t9*t10*t32*t564+t9*t10*t32*t566-t9*t10*t31*t568-t9*t10*t32*t568-t9*t10*t31*t574+t9*t10*t31*t575+t3*t4*t31*t588+t9*t10*t32*t575+t3*t4*t32*t588+t3*t4*t31*t592+t9*t10*t31*t580+t3*t4*t32*t592+t9*t10*t31*t582+t9*t10*t31*t584+t3*t4*t32*t609+t3*t4*t32*t610+t3*t4*t32*t612+t3*t4*t32*t613+t9*t10*t31*t605+t3*t4*t31*t624+t9*t10*t31*t621+t9*t10*t32*t621+t3*t4*t32*t659+t3*t4*t31*t663+t3*t4*t32*t667+t3*t4*t31*t670+t3*t4*t32*t670+t3*t4*t31*t672;
et8 = t3*t4*t31*t674+t3*t4*t31*t676+t3*t4*t31*t680+t3*t4*t31*t681+t3*t4*t32*t680+t3*t4*t32*t681+t9*t10*t31*t682+t3*t4*t31*t695*2.0+t9*t10*t31*t683+t9*t10*t32*t682+t3*t4*t32*t695+t9*t10*t32*t683-t3*t4*t31*t698*2.0+t3*t4*t32*t702-t9*t10*t31*t695*2.0-t9*t10*t32*t695+t3*t4*t31*t709+t3*t4*t32*t709+t9*t10*t31*t698*2.0+t9*t10*t32*t698+t9*t10*t32*t700-t9*t10*t32*t702+t3*t4*t31*t722+t3*t4*t32*t722+t9*t10*t31*t725+t3*t4*t32*t737+t3*t4*t31*t740+t3*t4*t32*t739+t3*t4*t32*t740+t3*t4*t31*t747+Lx2*Lycm2*m2*t3*t31+Lx2*Lycm3*m3*t3*t31+Lxcm2*Lycm2*m2*t3*t31+Lycm2*Lzcm2*m2*t9*t31+Lx4*t9*t11*t31*t55+Lx4*t9*t11*t32*t55;
et9 = -Lx4*t9*t11*t31*t59-Lx4*t9*t11*t31*t60-Lx4*t9*t11*t32*t59-Lx4*t9*t11*t31*t61-Lx4*t9*t11*t32*t60+Lx4*t9*t11*t33*t59-Lx4*t9*t11*t32*t61+Lx4*t9*t11*t33*t60+Lx4*t9*t11*t33*t61+Lx4*t9*t11*t31*t118+Lx4*t9*t11*t31*t119+Lx4*t9*t11*t32*t118+Lx4*t9*t11*t31*t120+Lx4*t9*t11*t32*t119+Lx4*t9*t11*t32*t120+Lx4*t9*t11*t34*t118+Lx4*t9*t11*t34*t119+Lx4*t9*t11*t34*t120-Lx4*t9*t11*t31*t131-Lx4*t9*t11*t32*t131+Lx4*t9*t11*t33*t131-Lx4*t9*t11*t34*t131+Lx4*t9*t11*t33*t143-Lx4*t9*t11*t31*t248-Lx4*t9*t11*t32*t248+Lx4*t9*t11*t33*t248-Lx4*t9*t11*t34*t248-Lx4*t9*t11*t35*t248+Lx4*t9*t11*t31*t257;
et10 = Lx4*t9*t11*t32*t257+Lx4*t9*t11*t34*t257+Lx4*t9*t11*t35*t257+Lx4*t9*t11*t33*t270+Lx4*t9*t11*t33*t271+Lx4*t9*t11*t33*t272+Lx4*t9*t11*t33*t429+Lxcm4*t9*t11*t31*t55+Lxcm4*t9*t11*t32*t55-Lxcm4*t9*t11*t31*t59-Lxcm4*t9*t11*t32*t59+Lxcm4*t9*t11*t33*t59-Lxcm4*t9*t11*t31*t127*2.0-Lxcm4*t9*t11*t32*t127*2.0+Lxcm4*t9*t11*t33*t143+Lycm4*t5*t9*t31*t55+Lycm4*t5*t9*t32*t55-Lycm4*t5*t9*t31*t59-Lycm4*t5*t9*t32*t59+Lycm4*t5*t9*t33*t59-Lycm5*t5*t9*t31*t60-Lycm5*t5*t9*t32*t60+Lycm5*t5*t9*t33*t60+Lycm5*t5*t9*t31*t119+Lycm5*t5*t9*t32*t119+Lycm5*t5*t9*t34*t119-Lycm5*t5*t9*t31*t131-Lycm5*t5*t9*t32*t131+Lycm5*t5*t9*t33*t131;
et11 = -Lycm5*t5*t9*t34*t131+Lycm4*t5*t9*t33*t143+Lycm5*t5*t9*t33*t271+t3*t4*t6*t31*t82-t3*t4*t6*t34*t82-t3*t4*t6*t31*t86+t3*t4*t6*t34*t86+t3*t10*t11*t31*t81+t4*t9*t11*t31*t81+t3*t10*t11*t32*t81+t4*t9*t11*t32*t81-t3*t10*t11*t33*t81-t4*t9*t11*t33*t81-t6*t9*t10*t31*t82+t3*t10*t11*t31*t85+t4*t9*t11*t31*t85+t6*t9*t10*t34*t82-t3*t10*t11*t33*t85-t4*t9*t11*t33*t85+t6*t9*t10*t31*t86-t6*t9*t10*t34*t86+t3*t10*t11*t33*t89+t4*t9*t11*t33*t89+t3*t10*t11*t33*t90+t4*t9*t11*t33*t90+t3*t4*t32*t45*t80-t9*t10*t32*t45*t80+t9*t10*t32*t44*t87+t9*t10*t32*t44*t88+t3*t10*t11*t31*t152;
et12 = t4*t9*t11*t31*t152+t3*t10*t11*t31*t153+t3*t10*t11*t32*t152+t4*t9*t11*t31*t153+t4*t9*t11*t32*t152+t3*t10*t11*t32*t153+t4*t9*t11*t32*t153+t3*t4*t32*t44*t150+t3*t4*t32*t44*t151+t9*t10*t31*t40*t150+t9*t10*t31*t40*t151-t3*t4*t6*t31*t287+t3*t4*t6*t34*t287+t3*t4*t6*t31*t291+t3*t10*t11*t31*t280+t3*t10*t11*t32*t280-t3*t4*t6*t34*t291+t3*t10*t11*t33*t285+t4*t9*t11*t33*t285+t6*t9*t10*t31*t287-t6*t9*t10*t34*t287+t3*t10*t11*t33*t290+t4*t9*t11*t33*t290-t6*t9*t10*t31*t291+t3*t10*t11*t31*t293+t4*t9*t11*t31*t293+t3*t10*t11*t32*t293+t4*t9*t11*t32*t293+t3*t10*t11*t31*t295-t3*t10*t11*t33*t293+t4*t9*t11*t31*t295;
et13 = -t4*t9*t11*t33*t293+t6*t9*t10*t34*t291+t3*t10*t11*t32*t295+t4*t9*t11*t32*t295+t3*t10*t11*t31*t297-t3*t10*t11*t33*t295+t4*t9*t11*t31*t297-t4*t9*t11*t33*t295+t3*t10*t11*t32*t297+t4*t9*t11*t32*t297-t3*t10*t11*t33*t297-t4*t9*t11*t33*t297+t3*t10*t11*t31*t304*2.0+t4*t9*t11*t31*t304*2.0+t3*t10*t11*t31*t305*2.0+t3*t10*t11*t32*t304+t4*t9*t11*t31*t305*2.0+t4*t9*t11*t32*t304+t3*t10*t11*t32*t305-t3*t10*t11*t33*t304*2.0+t4*t9*t11*t32*t305-t4*t9*t11*t33*t304*2.0+t3*t4*t32*t44*t279-t3*t10*t11*t33*t305*2.0-t4*t9*t11*t33*t305*2.0+t3*t10*t11*t31*t309+t4*t9*t11*t31*t309+t3*t10*t11*t32*t309+t4*t9*t11*t32*t309;
et14 = -t3*t10*t11*t33*t309-t4*t9*t11*t33*t309+t3*t10*t11*t33*t315+t4*t9*t11*t33*t315+t3*t4*t32*t44*t292+t3*t4*t32*t44*t294+t3*t4*t31*t41*t300*4.0+t3*t4*t32*t44*t296+t3*t4*t32*t41*t300+t9*t10*t32*t45*t286-t3*t10*t11*t31*t329*2.0-t4*t9*t11*t31*t329*2.0-t3*t10*t11*t31*t331*2.0+t3*t10*t11*t33*t329*2.0-t4*t9*t11*t31*t331*2.0+t4*t9*t11*t33*t329*2.0-t9*t10*t32*t44*t292+t3*t10*t11*t33*t331*2.0+t4*t9*t11*t33*t331*2.0+t3*t10*t11*t32*t333+t4*t9*t11*t32*t333-t9*t10*t32*t44*t294+t3*t10*t11*t32*t335+t4*t9*t11*t32*t335-t9*t10*t31*t41*t300*4.0-t9*t10*t32*t44*t296+t9*t10*t32*t45*t300-t3*t4*t32*t41*t326;
et15 = t9*t10*t32*t45*t312+t3*t4*t32*t45*t326-t3*t4*t6*t31*t374*2.0+t9*t10*t32*t41*t326-t3*t4*t6*t32*t374*2.0-t9*t10*t32*t45*t326+t3*t10*t11*t31*t445+t4*t9*t11*t31*t445+t3*t10*t11*t32*t445+t4*t9*t11*t32*t445+t3*t10*t11*t31*t449+t4*t9*t11*t31*t449+t3*t10*t11*t31*t472+t4*t9*t11*t31*t472+t3*t4*t32*t45*t446+t3*t10*t11*t32*t476+t4*t9*t11*t32*t476+t3*t10*t11*t32*t477+t4*t9*t11*t32*t477+t3*t10*t11*t32*t478+t4*t9*t11*t32*t478+t3*t10*t11*t32*t479+t4*t9*t11*t32*t479+t9*t10*t31*t41*t446+t3*t4*t32*t45*t461+t9*t10*t32*t41*t461+t3*t4*t32*t45*t470-t3*t4*t6*t31*t511*2.0-t6*t9*t10*t31*t499*2.0-t3*t4*t6*t31*t512*2.0-t3*t4*t6*t32*t511*2.0;
et16 = t6*t9*t10*t32*t499*-2.0-t3*t4*t6*t32*t512*2.0-t6*t9*t10*t31*t501*2.0-t6*t9*t10*t32*t501*2.0+t9*t10*t31*t41*t470+t3*t10*t11*t33*t571+t4*t9*t11*t33*t571+t3*t10*t11*t31*t577+t4*t9*t11*t31*t577+t3*t4*t32*t45*t574-t9*t10*t32*t45*t574+t3*t10*t11*t31*t668+t4*t9*t11*t31*t668+t3*t10*t11*t32*t668+t4*t9*t11*t32*t668+t3*t5*t10*t12*t31*t82+t4*t5*t9*t12*t31*t82+t3*t5*t10*t12*t32*t82+t4*t5*t9*t12*t32*t82-t3*t5*t10*t12*t33*t82-t4*t5*t9*t12*t33*t82+t3*t5*t10*t12*t34*t82+t4*t5*t9*t12*t34*t82-t3*t5*t10*t12*t31*t86-t4*t5*t9*t12*t31*t86-t3*t5*t10*t12*t32*t86-t4*t5*t9*t12*t32*t86;
et17 = t3*t5*t10*t12*t33*t86+t4*t5*t9*t12*t33*t86-t3*t5*t10*t12*t34*t86-t4*t5*t9*t12*t34*t86+t3*t10*t11*t32*t45*t85+t4*t9*t11*t32*t45*t85-t3*t5*t10*t12*t31*t287-t4*t5*t9*t12*t31*t287-t3*t5*t10*t12*t32*t287-t4*t5*t9*t12*t32*t287+t3*t5*t10*t12*t33*t287+t4*t5*t9*t12*t33*t287-t3*t5*t10*t12*t34*t287-t4*t5*t9*t12*t34*t287+t3*t5*t10*t12*t31*t291+t4*t5*t9*t12*t31*t291+t3*t5*t10*t12*t32*t291+t4*t5*t9*t12*t32*t291-t3*t5*t10*t12*t33*t291-t4*t5*t9*t12*t33*t291+t3*t5*t10*t12*t34*t291+t4*t5*t9*t12*t34*t291+t3*t10*t11*t33*t41*t449+t4*t9*t11*t33*t41*t449+t3*t10*t11*t32*t45*t449;
et18 = t4*t9*t11*t32*t45*t449+t9*t10*t31*t40*t41*t446+t9*t10*t32*t40*t41*t446+Lx2*Lx4*m4*t3*t11*t31+Lx2*Lx4*m5*t3*t11*t31-Lx2*Lx4*m4*t3*t11*t33+Lx2*Lx4*m6*t3*t11*t31-Lx2*Lx4*m5*t3*t11*t33-Lx2*Lx4*m6*t3*t11*t33+Lx2*Lxcm4*m4*t3*t11*t31-Lx2*Lxcm4*m4*t3*t11*t33+Lx3*Lycm3*m3*t3*t4*t31+Lx3*Lycm3*m3*t3*t4*t32+Lx2*Lycm4*m4*t3*t5*t31-Lx4*Lycm4*m4*t3*t4*t31-Lx2*Lycm4*m4*t3*t5*t33+Lx2*Lycm5*m5*t3*t5*t31-Lx4*Lycm5*m5*t3*t4*t31-Lx2*Lycm5*m5*t3*t5*t33+Lx4*Lycm4*m4*t9*t10*t31+Lx4*Lycm5*m5*t9*t10*t31+Lxcm3*Lycm3*m3*t3*t4*t31+Lxcm3*Lycm3*m3*t3*t4*t32-Lxcm4*Lycm4*m4*t3*t4*t31+Lxcm4*Lycm4*m4*t9*t10*t31+Lycm3*Lzcm3*m3*t3*t10*t31;
et19 = Lycm3*Lzcm3*m3*t3*t10*t32-Lxcm5*t6*t9*t11*t31*t60-Lxcm5*t6*t9*t11*t32*t60+Lxcm5*t6*t9*t11*t33*t60+Lxcm5*t6*t9*t11*t34*t60-Lxcm6*t5*t9*t13*t31*t61-Lxcm6*t5*t9*t13*t32*t61+Lxcm6*t5*t9*t13*t33*t61+Lxcm6*t5*t9*t13*t35*t61+Lxcm6*t5*t9*t13*t31*t118+Lxcm6*t5*t9*t13*t32*t118+Lxcm6*t5*t9*t13*t31*t120+Lxcm6*t5*t9*t13*t32*t120+Lxcm6*t5*t9*t13*t34*t118+Lxcm6*t5*t9*t13*t34*t120-Lxcm5*t6*t9*t11*t31*t128*2.0-Lxcm5*t6*t9*t11*t32*t128*2.0+Lxcm6*t5*t9*t13*t31*t256*2.0+Lxcm6*t5*t9*t13*t32*t256*2.0+Lxcm6*t5*t9*t13*t33*t270+Lxcm6*t5*t9*t13*t33*t272+Lxcm6*t5*t9*t13*t35*t270+Lxcm6*t5*t9*t13*t35*t272-Lycm6*t5*t7*t9*t31*t61-Lycm6*t5*t7*t9*t32*t61+Lycm6*t5*t7*t9*t33*t61;
et20 = Lycm6*t5*t7*t9*t35*t61+Lycm6*t5*t7*t9*t31*t118+Lycm6*t5*t7*t9*t32*t118+Lycm6*t5*t7*t9*t31*t120+Lycm6*t5*t7*t9*t32*t120+Lycm6*t5*t7*t9*t34*t118+Lycm6*t5*t7*t9*t34*t120+Lycm6*t5*t7*t9*t33*t270+Lycm6*t5*t7*t9*t33*t272+Lycm6*t5*t7*t9*t35*t270+Lycm6*t5*t7*t9*t35*t272-Lz6*t9*t11*t12*t31*t61-Lz6*t9*t11*t12*t32*t61+Lz6*t9*t11*t12*t33*t61+Lz6*t9*t11*t12*t34*t61-Lz6*t9*t11*t12*t31*t129*2.0-Lz6*t9*t11*t12*t32*t129*2.0-Lzcm5*t9*t11*t12*t31*t60-Lzcm5*t9*t11*t12*t32*t60+Lzcm5*t9*t11*t12*t33*t60-Lzcm6*t9*t11*t12*t31*t61+Lzcm5*t9*t11*t12*t34*t60-Lzcm6*t9*t11*t12*t32*t61+Lzcm6*t9*t11*t12*t33*t61+Lzcm6*t9*t11*t12*t34*t61+Lzcm6*t9*t11*t12*t31*t118*2.0;
et21 = Lzcm6*t9*t11*t12*t32*t118*2.0-Lzcm6*t9*t11*t12*t33*t118*2.0-Lzcm5*t9*t11*t12*t31*t128*2.0-Lzcm5*t9*t11*t12*t32*t128*2.0-Lzcm6*t9*t11*t12*t31*t129*2.0-Lzcm6*t9*t11*t12*t32*t129*2.0+Lx2*Lxcm5*m5*t3*t6*t11*t31-Lx2*Lxcm5*m5*t3*t6*t11*t33-Lx2*Lxcm5*m5*t3*t6*t11*t34+Lx2*Lxcm6*m6*t3*t5*t13*t31-Lx4*Lxcm6*m6*t3*t4*t13*t31-Lx2*Lxcm6*m6*t3*t5*t13*t33-Lx2*Lxcm6*m6*t3*t5*t13*t35-Lx4*Lxcm6*m6*t3*t4*t13*t35+Lx4*Lxcm6*m6*t9*t10*t13*t31+Lx4*Lxcm6*m6*t9*t10*t13*t35+Lx2*Lycm6*m6*t3*t5*t7*t31-Lx4*Lycm6*m6*t3*t4*t7*t31-Lx2*Lycm6*m6*t3*t5*t7*t33-Lx2*Lycm6*m6*t3*t5*t7*t35-Lx4*Lycm6*m6*t3*t4*t7*t35;
et22 = Lx4*Lycm6*m6*t7*t9*t10*t31+Lx4*Lycm6*m6*t7*t9*t10*t35+Lx4*Lycm4*m4*t3*t4*t31*t39*2.0+Lx4*Lycm4*m4*t3*t4*t32*t39+Lx4*Lycm5*m5*t3*t4*t31*t39*2.0+Lx4*Lycm5*m5*t3*t4*t32*t39-Lx4*Lycm4*m4*t3*t4*t32*t43-Lx4*Lycm5*m5*t3*t4*t32*t43-Lx4*Lycm4*m4*t9*t10*t31*t39*2.0-Lx4*Lycm4*m4*t9*t10*t32*t39-Lx4*Lycm5*m5*t9*t10*t31*t39*2.0-Lx4*Lycm5*m5*t9*t10*t32*t39+Lx4*Lycm4*m4*t9*t10*t32*t43+Lx4*Lycm5*m5*t9*t10*t32*t43-Lxcm5*Lycm5*m5*t3*t4*t6*t31+Lxcm5*Lycm5*m5*t3*t4*t6*t34+Lxcm6*Lycm6*m6*t3*t4*t6*t31-Lxcm6*Lycm6*m6*t3*t4*t6*t34+Lxcm5*Lycm5*m5*t6*t9*t10*t31-Lxcm5*Lycm5*m5*t6*t9*t10*t34-Lxcm6*Lycm6*m6*t6*t9*t10*t31+Lxcm6*Lycm6*m6*t6*t9*t10*t34;
et23 = Lxcm4*Lycm4*m4*t3*t4*t31*t39*2.0+Lxcm4*Lycm4*m4*t3*t4*t32*t39-Lxcm4*Lycm4*m4*t3*t4*t32*t43-Lxcm4*Lycm4*m4*t9*t10*t31*t39*2.0-Lxcm4*Lycm4*m4*t9*t10*t32*t39+Lxcm4*Lycm4*m4*t9*t10*t32*t43+Lx2*Lz6*m6*t3*t11*t12*t31-Lx2*Lz6*m6*t3*t11*t12*t33-Lx2*Lz6*m6*t3*t11*t12*t34+Lx4*Lzcm4*m4*t3*t10*t11*t31+Lx4*Lzcm4*m4*t3*t10*t11*t32+Lx2*Lzcm5*m5*t3*t11*t12*t31-Lx4*Lzcm4*m4*t3*t10*t11*t33-Lx2*Lzcm5*m5*t3*t11*t12*t33+Lx2*Lzcm6*m6*t3*t11*t12*t31-Lx2*Lzcm5*m5*t3*t11*t12*t34-Lx2*Lzcm6*m6*t3*t11*t12*t33-Lx2*Lzcm6*m6*t3*t11*t12*t34+Lxcm4*Lzcm4*m4*t3*t10*t11*t31+Lxcm4*Lzcm4*m4*t3*t10*t11*t32-Lxcm4*Lzcm4*m4*t3*t10*t11*t33;
et24 = -Lxcm5*Lzcm5*m5*t3*t10*t11*t31-Lxcm5*Lzcm5*m5*t4*t9*t11*t31+Lxcm5*Lzcm5*m5*t3*t10*t11*t33+Lxcm5*Lzcm5*m5*t4*t9*t11*t33+Lycm4*Lzcm4*m4*t3*t5*t10*t31+Lycm4*Lzcm4*m4*t3*t5*t10*t32-Lycm4*Lzcm4*m4*t3*t5*t10*t33-Lycm5*Lzcm5*m5*t3*t4*t12*t31+Lycm5*Lzcm5*m5*t3*t4*t12*t34+Lycm5*Lzcm5*m5*t9*t10*t12*t31-Lycm5*Lzcm5*m5*t9*t10*t12*t34-Lxcm6*t6*t7*t9*t11*t31*t61-Lxcm6*t6*t7*t9*t11*t32*t61+Lxcm6*t6*t7*t9*t11*t33*t61+Lxcm6*t6*t7*t9*t11*t34*t61+Lxcm6*t6*t7*t9*t11*t35*t61-Lxcm6*t6*t7*t9*t11*t31*t129*2.0-Lxcm6*t6*t7*t9*t11*t32*t129*2.0+Lxcm6*t5*t9*t13*t31*t40*t256*2.0+Lxcm6*t5*t9*t13*t32*t40*t256*2.0+Lycm6*t6*t9*t11*t13*t31*t61+Lycm6*t6*t9*t11*t13*t32*t61;
et25 = -Lycm6*t6*t9*t11*t13*t33*t61-Lycm6*t6*t9*t11*t13*t34*t61-Lycm6*t6*t9*t11*t13*t35*t61+Lycm6*t6*t9*t11*t13*t31*t129*2.0+Lycm6*t6*t9*t11*t13*t32*t129*2.0-t6*t9*t10*t11*t12*t31*t76*2.0-t6*t9*t10*t11*t12*t32*t76*2.0+t3*t6*t7*t10*t13*t31*t224*2.0+t4*t6*t7*t9*t13*t31*t224*2.0+t3*t6*t7*t10*t13*t32*t224*2.0+t4*t6*t7*t9*t13*t32*t224*2.0-t3*t6*t7*t10*t13*t33*t224*2.0-t4*t6*t7*t9*t13*t33*t224*2.0+Lx2*Lxcm6*m6*t3*t6*t7*t11*t31-Lx2*Lxcm6*m6*t3*t6*t7*t11*t33-Lx2*Lxcm6*m6*t3*t6*t7*t11*t34-Lx2*Lxcm6*m6*t3*t6*t7*t11*t35-Lx4*Lxcm5*m5*t3*t10*t11*t12*t31-Lx4*Lxcm5*m5*t3*t10*t11*t12*t32+Lx4*Lxcm5*m5*t3*t10*t11*t12*t33;
et26 = -Lx4*Lxcm5*m5*t3*t10*t11*t12*t34-Lx2*Lycm6*m6*t3*t6*t11*t13*t31+Lx2*Lycm6*m6*t3*t6*t11*t13*t33+Lx2*Lycm6*m6*t3*t6*t11*t13*t34+Lx2*Lycm6*m6*t3*t6*t11*t13*t35-Lxcm5*Lycm5*m5*t3*t5*t10*t12*t31-Lxcm5*Lycm5*m5*t3*t5*t10*t12*t32+Lxcm5*Lycm5*m5*t3*t5*t10*t12*t33-Lxcm5*Lycm5*m5*t3*t5*t10*t12*t34+Lxcm6*Lycm6*m6*t3*t5*t10*t12*t31+Lxcm6*Lycm6*m6*t4*t5*t9*t12*t31-Lxcm6*Lycm6*m6*t3*t5*t10*t12*t33-Lxcm6*Lycm6*m6*t4*t5*t9*t12*t33+Lxcm6*Lycm6*m6*t3*t5*t10*t12*t34+Lxcm6*Lycm6*m6*t4*t5*t9*t12*t34-Lxcm6*Lycm6*m6*t3*t4*t6*t31*t41*2.0+Lxcm6*Lycm6*m6*t3*t4*t6*t34*t41*2.0+Lxcm6*Lycm6*m6*t6*t9*t10*t31*t41*2.0-Lxcm6*Lycm6*m6*t6*t9*t10*t34*t41*2.0+Lx4*Lz6*m6*t3*t6*t10*t11*t31;
et27 = Lx4*Lz6*m6*t3*t6*t10*t11*t32-Lx4*Lz6*m6*t3*t6*t10*t11*t33+Lx4*Lz6*m6*t3*t6*t10*t11*t34+Lx4*Lzcm5*m5*t3*t6*t10*t11*t31+Lx4*Lzcm5*m5*t3*t6*t10*t11*t32-Lx4*Lzcm5*m5*t3*t6*t10*t11*t33+Lx4*Lzcm6*m6*t3*t6*t10*t11*t31+Lx4*Lzcm5*m5*t3*t6*t10*t11*t34+Lx4*Lzcm6*m6*t3*t6*t10*t11*t32-Lx4*Lzcm6*m6*t3*t6*t10*t11*t33+Lx4*Lzcm6*m6*t3*t6*t10*t11*t34-Lxcm6*Lz6*m6*t3*t7*t10*t11*t31-Lxcm6*Lz6*m6*t4*t7*t9*t11*t31+Lxcm6*Lz6*m6*t3*t7*t10*t11*t33+Lxcm6*Lz6*m6*t4*t7*t9*t11*t33-Lxcm6*Lz6*m6*t3*t7*t10*t11*t35-Lxcm6*Lz6*m6*t4*t7*t9*t11*t35-Lxcm6*Lzcm6*m6*t3*t7*t10*t11*t31-Lxcm6*Lzcm6*m6*t4*t7*t9*t11*t31+Lxcm6*Lzcm6*m6*t3*t7*t10*t11*t33;
et28 = Lxcm6*Lzcm6*m6*t4*t7*t9*t11*t33-Lxcm6*Lzcm6*m6*t3*t7*t10*t11*t35-Lxcm6*Lzcm6*m6*t4*t7*t9*t11*t35+Lxcm5*Lzcm5*m5*t3*t10*t11*t31*t40*2.0+Lxcm5*Lzcm5*m5*t4*t9*t11*t31*t40*2.0+Lxcm5*Lzcm5*m5*t3*t10*t11*t32*t40+Lxcm5*Lzcm5*m5*t4*t9*t11*t32*t40-Lxcm5*Lzcm5*m5*t3*t10*t11*t33*t40*2.0-Lxcm5*Lzcm5*m5*t4*t9*t11*t33*t40*2.0-Lxcm5*Lzcm5*m5*t3*t10*t11*t32*t44-Lxcm5*Lzcm5*m5*t4*t9*t11*t32*t44+Lycm6*Lz6*m6*t3*t10*t11*t13*t31+Lycm6*Lz6*m6*t4*t9*t11*t13*t31-Lycm6*Lz6*m6*t3*t10*t11*t13*t33-Lycm6*Lz6*m6*t4*t9*t11*t13*t33+Lycm6*Lz6*m6*t3*t10*t11*t13*t35+Lycm6*Lz6*m6*t4*t9*t11*t13*t35+Lycm5*Lzcm5*m5*t3*t5*t6*t10*t31+Lycm5*Lzcm5*m5*t3*t5*t6*t10*t32-Lycm5*Lzcm5*m5*t3*t5*t6*t10*t33;
et29 = Lycm5*Lzcm5*m5*t3*t5*t6*t10*t34+Lycm6*Lzcm6*m6*t3*t10*t11*t13*t31+Lycm6*Lzcm6*m6*t4*t9*t11*t13*t31-Lycm6*Lzcm6*m6*t3*t10*t11*t13*t33-Lycm6*Lzcm6*m6*t4*t9*t11*t13*t33+Lycm6*Lzcm6*m6*t3*t10*t11*t13*t35+Lycm6*Lzcm6*m6*t4*t9*t11*t13*t35-Lz6*Lzcm6*m6*t5*t9*t10*t11*t31*2.0-Lx4*Lxcm6*m6*t3*t7*t10*t11*t12*t31-Lx4*Lxcm6*m6*t3*t7*t10*t11*t12*t32+Lx4*Lxcm6*m6*t3*t7*t10*t11*t12*t33-Lx4*Lxcm6*m6*t3*t7*t10*t11*t12*t34-Lx4*Lxcm6*m6*t3*t7*t10*t11*t12*t35+Lx4*Lycm6*m6*t3*t10*t11*t12*t13*t31+Lx4*Lycm6*m6*t3*t10*t11*t12*t13*t32-Lx4*Lycm6*m6*t3*t10*t11*t12*t13*t33+Lx4*Lycm6*m6*t3*t10*t11*t12*t13*t34+Lx4*Lycm6*m6*t3*t10*t11*t12*t13*t35-Lxcm6*Lycm6*m6*t3*t5*t10*t12*t31*t41*2.0;
et30 = Lxcm6*Lycm6*m6*t4*t5*t9*t12*t31*t41*-2.0-Lxcm6*Lycm6*m6*t3*t5*t10*t12*t32*t41-Lxcm6*Lycm6*m6*t4*t5*t9*t12*t32*t41+Lxcm6*Lycm6*m6*t3*t5*t10*t12*t33*t41*2.0+Lxcm6*Lycm6*m6*t4*t5*t9*t12*t33*t41*2.0-Lxcm6*Lycm6*m6*t3*t5*t10*t12*t34*t41*2.0-Lxcm6*Lycm6*m6*t4*t5*t9*t12*t34*t41*2.0+Lxcm6*Lycm6*m6*t3*t5*t10*t12*t32*t45+Lxcm6*Lycm6*m6*t4*t5*t9*t12*t32*t45+Lxcm6*Lz6*m6*t3*t5*t6*t10*t13*t31+Lxcm6*Lz6*m6*t3*t5*t6*t10*t13*t32-Lxcm6*Lz6*m6*t3*t5*t6*t10*t13*t33+Lxcm6*Lz6*m6*t3*t5*t6*t10*t13*t34-Lxcm6*Lz6*m6*t3*t5*t6*t10*t13*t35+Lxcm6*Lzcm6*m6*t3*t5*t6*t10*t13*t31+Lxcm6*Lzcm6*m6*t3*t5*t6*t10*t13*t32-Lxcm6*Lzcm6*m6*t3*t5*t6*t10*t13*t33+Lxcm6*Lzcm6*m6*t3*t5*t6*t10*t13*t34;
et31 = -Lxcm6*Lzcm6*m6*t3*t5*t6*t10*t13*t35+Lycm6*Lz6*m6*t3*t5*t6*t7*t10*t31+Lycm6*Lz6*m6*t3*t5*t6*t7*t10*t32-Lycm6*Lz6*m6*t3*t5*t6*t7*t10*t33+Lycm6*Lz6*m6*t3*t5*t6*t7*t10*t34-Lycm6*Lz6*m6*t3*t5*t6*t7*t10*t35+Lycm6*Lzcm6*m6*t3*t5*t6*t7*t10*t31+Lycm6*Lzcm6*m6*t3*t5*t6*t7*t10*t32-Lycm6*Lzcm6*m6*t3*t5*t6*t7*t10*t33+Lycm6*Lzcm6*m6*t3*t5*t6*t7*t10*t34-Lycm6*Lzcm6*m6*t3*t5*t6*t7*t10*t35-Lz6*Lzcm6*m6*t3*t6*t10*t11*t12*t33*2.0-Lz6*Lzcm6*m6*t5*t9*t10*t11*t32*t44*2.0-Lxcm6*Lycm6*m6*t3*t4*t5*t7*t11*t13*t31*2.0-Lxcm6*Lycm6*m6*t3*t4*t5*t7*t11*t13*t32*2.0;
et32 = -t34*(-t71-t73-t74+t102-t172-t174-t176+t200+t203+t206-t222-t223+t224+t348+t353+t354+t357-t375+t378+t379+t380+t381+t383+t387-t388+t486-t567-t593+t594+t632+Lx2*t131+Lx2*t248+Lx2*t270+Lx2*t271+Lx2*t272+Lx2*t429)+t30*(t598+t599+t656+t715+t717+t718+t797+t798+t799+t829+t830-(Ixx2*t42)./2.0+(Izz2*t42)./2.0+m3*t2*t761*t828+m3*t8*t761*t825-m5*t2*t831*t853+m4*t2*t837*t851+m5*t8*t831*t852+m4*t8*t837*t848-m6*t2*t850*t860+m6*t8*t850*t857+m2*t2*t691*(t65-Lycm2*t8+Lxcm2*t2*t3+Lzcm2*t2*t9)+m2*t8*t691*(t91+Lycm2*t2+Lxcm2*t3*t8+Lzcm2*t8*t9));
et33 = -t33*(t72+t75+t148+t155+t172+t174+t176+t182+t183+t204+t207+t223+t348+t375+t378+t379+t380+t388+t403+t404+t405+t406+t407+t408+t415+t425+t435+t441+t442+t443+t486+t523+t524+t526+t541+t543+t547+t554+t567+t593+t595+t596+t601+t602+t632+t660+t661+t662+t678+t689+t697+t735+Lx2*t127+Lx2*t128+Lx2*t129+Lx2*t130+Lx2*t275+Lx2*t276+Lx2*t428+Lx2*t433)-Lx2*t32*t856+m6*t35*(t113+t114+t117+t236+t237+t239+t240+t241+t265+t266+t269+t423-Lx2*Lxcm6*t4*t7*t12+Lx2*Lxcm6*t10*t11*t13+Lx2*Lycm6*t7*t10*t11+Lx2*Lycm6*t4*t12*t13-Lx2*Lxcm6*t5*t6*t7*t10+Lx2*Lycm6*t5*t6*t10*t13);
et34 = t83*t109+t84*t109+t109*t149+Ixx6*(t262-t754)*(t5*t13*t52+t7*t11*t122)+m4*(-Lycm4*t764+Lx4*(t53-t759)+Lxcm4*(t53-t759))*(t91+t753+t769+Lxcm4*t764+Lzcm4*t690+Lycm4*(t53-t759))+m6*t858*(-Lycm6*(t7*t764+t6*t13*(t53-t759))+Lx4*(t53-t759)-Lxcm6*(t13*t764+t6*t789)+Lz6*t12*(t53-t759)+Lzcm6*t12*(t53-t759))-m4*(t766+Lxcm4*t762-Lycm4*(t63-t756))*(t65+t750+t778-Lycm4*t762+Lzcm4*t688-Lxcm4*(t63-t756))-m5*t855*(t766-Lycm5*(t63-t756)+Lxcm5*t6*t762+Lzcm5*t12*t762);
et35 = m5*t854*(-Lycm5*t764+Lx4*(t53-t759)+Lxcm5*t6*(t53-t759)+Lzcm5*t12*(t53-t759))-m6*t859*(t766+Lxcm6*(t6*t774-t13*(t63-t756))-Lycm6*(t6*t776+t7*(t63-t756))+Lz6*t12*t762+Lzcm6*t12*t762)+Iyy6*t782*(t5*t7*t52-t11*t13*t122)-Ixx5*t11*t122*t728+Izz5*t11*t132*t751+Izz6*t11*t132*t751;
et36 = -t30*(et34+et35)+t31*(t69+t70+t80+t83+t84+t98+t99+t100+t101+t149+t150+t151+t159+t160+t161+t170+t199+t201+t225+t226+t227+t278+t279+t281+t282+t283+t284+t292+t294+t296+t298+t299+t313+t318+t320+t323+t326+t330+t351+t434+t436+t437+t438+t446+t447+t448+t455+t456+t461+t466+t468+t470+t474+t475+t489+t490+t538+t558+t561+t562+t564+t568+t570+t574+t588+t592+t609+t610+t612+t613+t624+t633+t634+t659+t663+t667+t670+t672+t674+t676+t680+t681+t686+t695+t702+t705+t706+t709+t712+t722+t737+t739+t740+t747+Lx2*Lx4*m4*t4*t11+Lx2*Lx4*m5*t4*t11+Lx2*Lx4*m6*t4*t11+Lx2*Lxcm4*m4*t4*t11+Lx2*Lycm4*m4*t4*t5+Lx2*Lycm5*m5*t4*t5+Lx2*Lxcm5*m5*t4*t6*t11+Lx2*Lxcm6*m6*t4*t5*t13+Lx2*Lycm6*m6*t4*t5*t7+Lx2*Lz6*m6*t4*t11*t12+Lx2*Lzcm5*m5*t4*t11*t12+Lx2*Lzcm6*m6*t4*t11*t12+Lx2*Lxcm6*m6*t4*t6*t7*t11-Lx2*Lycm6*m6*t4*t6*t11*t13);
et37 = -t35*(t205+t208+t228+t229+Lx4*Lxcm6*m6*t13+Lx4*Lycm6*m6*t7)+t32*(t69+t70+t80+t83+t84+t98+t99+t100+t101+t149+t150+t151+t159+t160+t161+t170+t199+t201+t225+t226+t227+t278+t279+t281+t282+t283+t284+t292+t294+t296+t298+t299+t313+t318+t320+t323+t326+t330+t351+t434+t436+t437+t438+t446+t447+t448+t455+t456+t461+t466+t468+t470+t474+t475+t489+t490+t538+t558+t561+t562+t564+t568+t570+t574+t588+t592+t609+t610+t612+t613+t624+t633+t634+t659+t663+t667+t670+t672+t674+t676+t680+t681+t686+t695+t702+t705+t706+t709+t712+t722+t737+t739+t740+t747)+t34*(t205+t208+t228+t229-t6*t82+t6*t86+t6*t287-t6*t291+Lxcm5*Lycm5*m5*t6-Lxcm6*Lycm6*m6*t6+Lycm5*Lzcm5*m5*t12+Lxcm6*Lycm6*m6*t6*t41*2.0);
et38 = -t33*(t81+t85+t152+t153+t163+t280+t293+t295+t297+t304+t305+t309+t333+t335+t445+t449+t472+t476+t477+t478+t479+t577+t591+t668-Lx4*Lxcm5*m5*t12+Lx4*Lz6*m6*t6+Lx4*Lzcm5*m5*t6+Lx4*Lzcm6*m6*t6-Lx4*Lxcm6*m6*t7*t12+Lx4*Lycm6*m6*t12*t13)+t32*(t81+t85+t152+t153+t163+t198+t280+t293+t295+t297+t304+t305+t309+t319+t321+t322+t333+t335+t350+t356+t377+t400+t401+t402+t445+t449+t462+t463+t464+t467+t471+t472+t476+t477+t478+t479+t487+t488+t498+t500+t502+t532+t537+t540+t560+t569+t576+t577+t591+t608+t625+t628+t629+t630+t631+t635+t647+t664+t668+t673+t675+t677+t685+t707+t708+t710+t713+t714+t720+t723+t730+t741+t748);
et39 = t31*(t81+t85+t152+t153+t163+t198+t280+t293+t295+t297+t304+t305+t309+t319+t321+t322+t333+t335+t350+t356+t377+t400+t401+t402+t445+t449+t462+t463+t464+t467+t471+t472+t476+t477+t478+t479+t487+t488+t498+t500+t502+t532+t537+t540+t560+t569+t576+t577+t591+t608+t625+t628+t629+t630+t631+t635+t647+t664+t668+t673+t675+t677+t685+t707+t708+t710+t713+t714+t720+t723+t730+t741+t748+Lx2*t5*t131+Lx2*t5*t248+Lx2*t5*t270+Lx2*t5*t271+Lx2*t5*t272+Lx2*t5*t429+Lx2*Lxcm5*m5*t6*t10+Lx2*Lz6*m6*t10*t12+Lx2*Lzcm5*m5*t10*t12+Lx2*Lzcm6*m6*t10*t12+Lx2*Lxcm6*m6*t6*t7*t10-Lx2*Lycm6*m6*t6*t10*t13);
et40 = t30*(m6*t858*(Lz6*t808+Lzcm6*t808+Lxcm6*t7*t806-Lycm6*t13*t806)+m6*t859*(Lz6*t817+Lzcm6*t817+Lxcm6*t7*t812-Lycm6*t13*t812)-Ixx5*t728*t751+Izz5*t728*t751+Izz6*t728*t751+m5*t854*(Lxcm5*t806+Lzcm5*t808)+m5*t855*(Lxcm5*t812+Lzcm5*t817)-Iyy6*t13*t751*t782+Ixx6*t7*t751*(t262-t754))-m6*t35*(Lxcm6*t7-Lycm6*t13)*(Lz6+Lzcm6);
et41 = t34*(-t82+t86+t162+t287-t291)+t32*(t202+t311+t316+t338+t349+t352+t414+t469+t473+t499+t501+t519+t525+t527+t531+t539+t542+t544+t552+t556+t559+t563+t572+t579+t626+t642+t643+t646+t649+t652+t653+t654+t655+t658+t666+t669+t671+t693+t701+t703+t711+t716+t724+t736+t738+t745+t749)-t30*(m6*t859*(Lycm6*t838-Lxcm6*(t774-t822))+m6*t858*(Lxcm6*t842+Lycm6*(t818-t13*(t53-t759)))+Ixx6*t782*(t262-t754)-Iyy6*t782*(t262-t754))+t33*(t82-t86-t162-t287+t291-t311+t317+t355+t358+t382+t384+t520-t531+t573-t579+Lx4*Lxcm6*m6*t6*t13+Lx4*Lycm6*m6*t6*t7);
et42 = t31*(t202+t311+t316+t338+t349+t352+t414+t469+t473+t499+t501+t519+t525+t527+t531+t539+t542+t544+t552+t556+t559+t563+t572+t579+t626+t642+t643+t646+t649+t652+t653+t654+t655+t658+t666+t669+t671+t693+t701+t703+t711+t716+t724+t736+t738+t745+t749+Lx2*Lxcm6*m6*t4*t7*t11-Lx2*Lxcm6*m6*t10*t12*t13-Lx2*Lycm6*m6*t4*t11*t13-Lx2*Lycm6*m6*t7*t10*t12+Lx2*Lxcm6*m6*t4*t5*t6*t13+Lx2*Lycm6*m6*t4*t5*t6*t7);
mt1 = [et1+et2+et3+et4+et5+et6+et7+et8+et9+et10+et11+et12+et13+et14+et15+et16+et17+et18+et19+et20+et21+et22+et23+et24+et25+et26+et27+et28+et29+et30+et31;et32+et33;-t33*(t72+t75+t148+t155+t172+t174+t176+t182+t183+t204+t207+t223+t375+t388+t403+t404+t405+t406+t407+t408+t415+t425+t435+t441+t442+t443+t523+t524+t526+t541+t543+t547+t554+t567+t593+t595+t596+t601+t602+t660+t661+t662+t678+t689+t697+t735)+t30*(t598+t599+t656+t715+t717+t718+t797+t798+t799+t829+t830+m3*t2*t760*t828+m3*t8*t760*t825-m5*t2*t826*t853+m5*t8*t826*t852+m4*t2*t835*t851+m4*t8*t835*t848-m6*t2*t849*t860+m6*t8*t849*t857)+t34*(t71+t73+t74-t102+t172+t174+t176-t203+t222+t223+t375+t388+t407+t408+t415+t523+t524+t526+t541+t543+t547+t567+t593+t689)+m6*t35*(t113+t114+t117+t236+t237+t239+t240+t241+t265+t266+t269+t423)+Lx2*t31*t856];
mt2 = [et36+et37;et38+et39+et40;et41+et42];
out1 = [mt1;mt2];
end
